simulink model "LADRC3"  (R2023a)
settings: Solver=VariableStepAuto  StartTime=0.0  StopTime=20  FixedStep=0.001  RelTol=1e-3
settings Model: Creator=belov  LastModifiedBy=belov

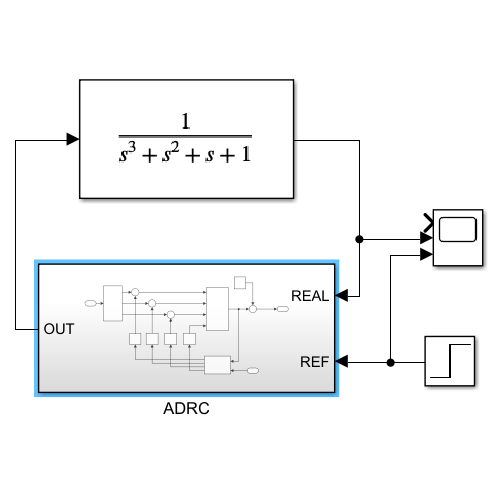
[thumbnail: Simulink's stored preview of the top-level diagram]
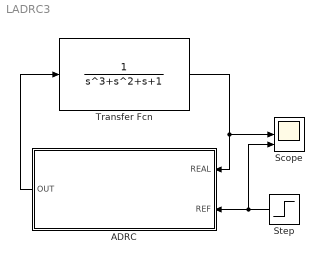
== system LADRC3 ==
  ADRC : Subsystem
  Scope : Scope  NumInputPorts=3
  Step : Step  SampleTime=0
  Transfer Fcn : TransferFcn  Denominator=[1 1 1 1]
  wires:
  Transfer Fcn/1 -> ADRC/1(REAL), Scope/2
  ADRC/1(OUT) -> Transfer Fcn/1
  Step/1 -> ADRC/2(REF), Scope/3

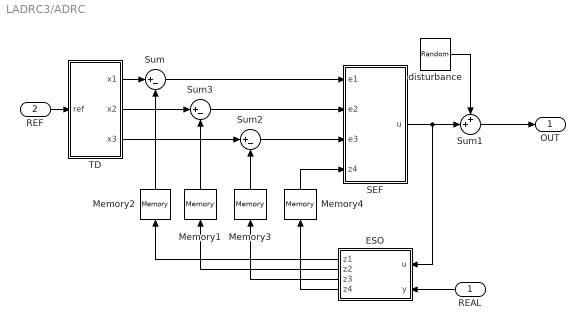
== system LADRC3/ADRC ==
  REAL : Inport
  REF : Inport  Port=2
  ESO : MATLAB Function  TreatAsAtomicUnit=on  SystemSampleTime=0.001
  Memory{1..4} (4 alike) : Memory
  SEF : MATLAB Function  TreatAsAtomicUnit=on  SystemSampleTime=0.001
  Sum : Sum  Inputs=|+-
  Sum1 : Sum  Inputs=++|
  Sum2 : Sum  Inputs=|+-
  Sum3 : Sum  Inputs=|+-
  TD : MATLAB Function  TreatAsAtomicUnit=on  SystemSampleTime=0.001
  disturbance : UniformRandomNumber  SampleTime=0.1
  OUT : Outport
  wires:
  REAL/1 -> ESO/2(y)
  TD/1(x1) -> Sum/1
  Sum/1 -> SEF/1(e1)
  TD/2(x2) -> Sum3/1
  TD/3(x3) -> Sum2/1
  Sum3/1 -> SEF/2(e2)
  Sum2/1 -> SEF/3(e3)
  ESO/1(z1) -> Memory2/1
  ESO/2(z2) -> Memory1/1
  ESO/3(z3) -> Memory3/1
  ESO/4(z4) -> Memory4/1
  Memory2/1 -> Sum/2
  Memory1/1 -> Sum3/2
  Memory3/1 -> Sum2/2
  Memory4/1 -> SEF/4(z4)
  REF/1 -> TD/1(ref)
  SEF/1(u) -> Sum1/2, ESO/1(u)
  disturbance/1 -> Sum1/1
  Sum1/1 -> OUT/1

== matlab function LADRC3/ADRC/SEF ==
  data: e1 input; u output; e2 input; e3 input; z4 input
function u = SEF(e1, e2, e3, z4)

b0 = 1;

wc = 50;

a1 = wc * wc * wc;
a2 = 3 * wc * wc;
a3 = 3 * wc;
u0 = a1 * e1 + a2 * e2 + a3 * e3;
u = (u0 - z4) / b0;
% u = 1 / b0 * (a1 * e1 + a2 * e2 + a3 * e3 + z4);

end

== matlab function LADRC3/ADRC/TD ==
  data: ref input; x1 output; x2 output; x3 output
function [x1, x2, x3] = TD(ref)

persistent x1_ x2_ x3_;

h = 0.001; % 步长
r = 10;

if isempty(x1_)
    x1_=0;
end
if isempty(x2_)
    x2_=0;
end
if isempty(x3_)
    x3_=0;
end

x1 = x1_ + h * x2_;
x2 = x2_ + h * x3_;
x3 = x3_ - h * (3 * r * x3_ + 3 * r * r * x2_ + r * r * r * x1_ - r * r * r * ref);

x1_ = x1;
x2_ = x2;
x3_ = x3;
end

== matlab function LADRC3/ADRC/ESO ==
  data: u input; z1 output; y input; z2 output; z3 output; z4 output
function [z1, z2, z3, z4] = ESO(u, y)

wo = 250;
b0 = 1;

beta1 = 4 * wo;
beta2 = 6 * wo * wo;
beta3 = 4 * wo * wo * wo;
beta4 = wo * wo * wo * wo;

h = 0.001;

persistent z1_ z2_ z3_ z4_;

if isempty(z1_)
    z1_ = 0;
end
if isempty(z2_)
    z2_ = 0;
end
if isempty(z3_)
    z3_ = 0;
end
if isempty(z4_)
    z4_ = 0;
end
z1 = z1_ + h * (-beta1 * z1_ + z2_ + beta1 * y);
z2 = z2_ + h * (-beta2 * z1_ + z3_ + beta2 * y);
z3 = z3_ + h * (-beta3 * z1_ + z4_ + b0 * u + beta3 * y);
z4 = z4_ + h * (-beta4 * z1_ + beta4 * y);

z1_ = z1;
z2_ = z2;
z3_ = z3;
z4_ = z4;
end
